simulink model "UAVSlung2"  (R2023a)
settings: Solver=ode45  StartTime=0.0  StopTime=16  RelTol=1e-4
values from neighbouring files (symbols this model uses):
  x0 = [0.1 -0.1 0 0 0 -0.5 2 0 0 0 0 0 0 0 0 0 0 0 0]    [main.m]
settings Model: Creator=KANG  LastModifiedBy=kang
settings DataIOCC: ReturnWorkspaceOutputs=off  TimeSaveName=tout1
settings DebuggingCC: UnconnectedInputMsg=warning  UnconnectedOutputMsg=warning  UnconnectedLineMsg=warning
settings ModelReferenceCC: EnableRefExpFcnMdlSchedulingChecks=on
settings RTWCC: DLArmComputeVersion=19.05

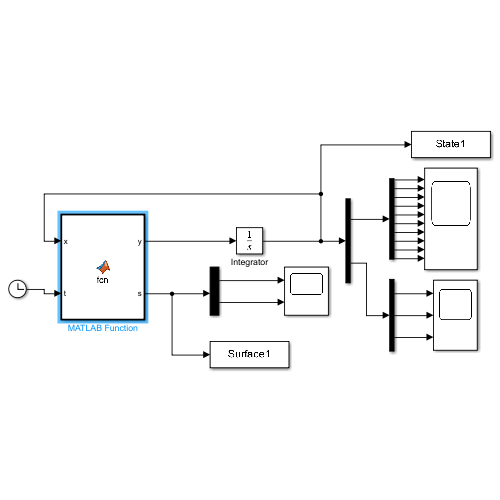
[thumbnail: Simulink's stored preview of the top-level diagram]
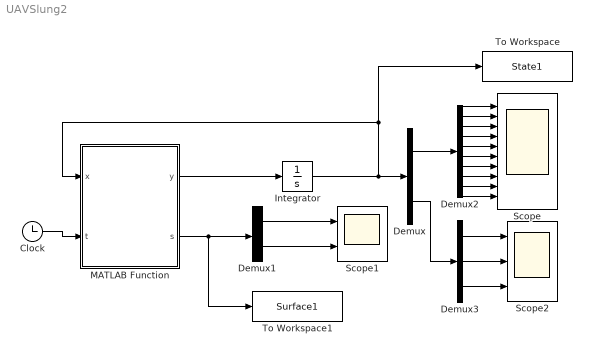
== system UAVSlung2 ==
  Clock : Clock
  Demux : Demux  Outputs=[10,9]
  Demux1 : Demux  Outputs=2
  Demux2 : Demux  Outputs=10
  Demux3 : Demux  Outputs=[-1,-1,-1]
  Integrator : Integrator  InitialCondition=x0
  MATLAB Function : MATLAB Function  TreatAsAtomicUnit=on
  Scope : Scope  NumInputPorts=10
  Scope1 : Scope  NumInputPorts=2
  Scope2 : Scope  NumInputPorts=3
  To Workspace : ToWorkspace  VariableName=State1  SaveFormat=Structure With Time  SampleTime=-1
  To Workspace1 : ToWorkspace  VariableName=Surface1  SaveFormat=Structure With Time  SampleTime=-1
  wires:
  MATLAB Function/1(y) -> Integrator/1
  Clock/1 -> MATLAB Function/2(t)
  MATLAB Function/2(s) -> To Workspace1/1, Demux1/1
  Integrator/1 -> To Workspace/1, MATLAB Function/1(x), Demux/1
  Demux/1 -> Demux2/1
  Demux1/1 -> Scope1/1
  Demux1/2 -> Scope1/2
  Demux2/1 -> Scope/1
  Demux2/2 -> Scope/2
  Demux2/3 -> Scope/3
  Demux2/4 -> Scope/4
  Demux2/5 -> Scope/5
  Demux2/6 -> Scope/6
  Demux2/7 -> Scope/7
  Demux2/8 -> Scope/8
  Demux2/9 -> Scope/9
  Demux2/10 -> Scope/10
  Demux3/1 -> Scope2/1
  Demux3/2 -> Scope2/2
  Demux/2 -> Demux3/1
  Demux3/3 -> Scope2/3

== matlab function UAVSlung2/MATLAB Function ==
  data: x input; y output; t input; s output
function [y, s] = fcn(x, t)
y=zeros(19,1);
s=zeros(9,1);
%% 
%  1-4 theta1 theta2 dtheta1 dtheta2
%  
%  5-10 x y z dx dy dz
%% 
l=0.5; g=9.81; mp=0.5;mq=1.121;
m=mp+mq;


% %% M ,C  G   u 
% M=zeros(5,5);
% M(1,1)=mq+mp;M(2,2)=mq+mp;M(3,3)=mq+mp;M(4,4)=mp*l^2*cos(x(2))^2;M(5,5)=mp*l^2;
% M(1,4)=mp*l*cos(x(1))*cos(x(2));
% M(4,1)=M(1,4);
% M(1,5)=-mp*l*sin(x(1))*sin(x(2));
% M(5,1)=M(1,5);
% M(2,5)=mp*l*cos(x(2));
% M(5,2)=M(2,5);
% M(3,4)=mp*l*sin(x(1))*cos(x(2));
% M(4,3)=M(3,4);
% M(3,5)=mp*l*cos(x(1))*sin(x(2));
% M(5,3)=M(3,5);
% % 
% 
% C=zeros(5,5);
% 
% C(1,4)=-mp*l*x(3)*sin(x(1))*cos(x(2))-mp*l*x(4)*cos(x(1))*sin(x(2));
% C(1,5)=-mp*l*x(3)*cos(x(1))*sin(x(2))-mp*l*x(4)*sin(x(1))*cos(x(2));
% C(2,5)=-mp*l*x(4)*sin(x(2));
% C(3,4)=mp*l*x(3)*cos(x(1))*cos(x(2))-mp*l*x(4)*sin(x(1))*sin(x(2));
% C(3,5)=-mp*l*x(3)*sin(x(1))*sin(x(2))+mp*l*x(4)*cos(x(1))*cos(x(2));
% C(4,4)=-mp*l^2*x(4)*cos(x(2))*sin(x(2));
% C(4,5)=-mp*l^2*x(3)*cos(x(2))*sin(x(2));
% C(5,4)=mp*l^2*x(3)*cos(x(2))*sin(x(2));
% 
% G=[0 0 0 mp*g*l*sin(x(1))*cos(x(2)) mp*g*l*cos(x(1))*sin(x(2))]';




e3=[0 0 1]';


%%

rd=[1,0.5,3];% target point

c11=0.6;c21=0.6;c31=0.6; c12=0;c22=0;c32=0; % gains for sliding mode manifold 

Sx=c11*(x(5)-rd(1))+x(8)-c12*sin(x(1))*cos(x(2));
Sy=c21*(x(6)-rd(2))+x(9)-c22*sin(x(2));
Sz=c31*(x(7)-rd(3))+x(10)+c32-c32*cos(x(1))*cos(x(2));

d=0.1*[1*sin(t),2*sin(t),1*sin(t)]';  % disturbances



k11=0;k21=0;k31=0; k12=2;k22=2;k32=2;% control gains
%% controller
vx1=-k11*(Sx)-k12*sig(Sx,0.5)+1*x(11)-x(17);
vy1=-k21*(Sy)-k22*sig(Sy,0.5)+1*x(12)-x(18);
vz1=-k31*(Sz)-k32*sig(Sz,0.5)+1*x(13)-x(19);

vx=-c11*x(8)+c12*(cos(x(1))*cos(x(2))*x(3)-sin(x(1))*sin(x(2))*x(4))+vx1;
vy=-c21*x(9)+c22*cos(x(2))*x(4)+vy1;
vz=-c31*x(10)-c32*(sin(x(1))*cos(x(2))*x(3)+cos(x(1))*sin(x(2))*x(4))+vz1;


%*******
%  11-13 super twisting controller
y(11)=-1*sign(Sx);
y(12)=-1*sign(Sy);
y(13)=-1*sign(Sz);

%% super twisting observer 
%14-16 estimation of sliding manifold
%17-19 estimation of disturbance

lam1=-1.5*5^0.5*sig(x(14)-Sx,0.5)+x(17);
lam2=-1.5*5^0.5*sig(x(15)-Sy,0.5)+x(18);
lam3=-1.5*5^0.5*sig(x(16)-Sz,0.5)+x(19);

y(14)=vx+lam1;
y(15)=vy+lam2;
y(16)=vz+lam3;



y(17)=-1.1*5*sign(x(17)-lam1);
y(18)=-1.1*5*sign(x(18)-lam2);
y(19)=-1.1*5*sign(x(19)-lam3);


M1=[m-mp+mp*sin(x(1))^2*cos(x(2))^2,mp*sin(x(1))*sin(x(2))*cos(x(2)),-mp*sin(x(1))*cos(x(1))*cos(x(2))^2;...
    mp*sin(x(1))*sin(x(2))*cos(x(2)),m-mp*cos(x(2))^2,-mp*sin(x(2))*cos(x(1))*cos(x(2));...
    -mp*sin(x(1))*cos(x(1))*cos(x(2))^2,-mp*sin(x(2))*cos(x(1))*cos(x(2)),m-mp+mp*cos(x(1))^2*cos(x(2))^2];

y(5:7)=x(8:10); 

y(8:10)=[vx;vy;vz]+M1\d;


% f=[-mp*l*(sin(u(1))*cos(u(2))*u(3)^2+2*sin(u(2))*cos(u(1))*u(3)*u(4)+sin(u(1))*sin(u(2))*u(4)^2);...
%    -mp*l*(sin(u(2))*u(4)^2;...
%     mp*l*(cos(u(1))*cos(u(2))*u(3)^2-2*sin(u(2))*sin(u(1))*u(3)*u(4)+cos(u(1))*cos(u(2))*u(4)^2)];

f=[mp*(-g*sin(x(1))*cos(x(1))*cos(x(2))^3-sin(x(1))*cos(x(2))*l*x(3)^2-sin(x(1))*sin(x(2))*l*x(4)^2);...
   mp*(-l*cos(x(2))^2*x(3)^2-g*cos(x(1))*cos(x(2))-l*x(4)^2)*sin(x(2));...
   mp*(-g+g*cos(x(1))^2*cos(x(2))^2+l*cos(x(1))*cos(x(2))^3*x(3)^2+l*cos(x(1))*cos(x(2))*x(4)^2)];
%%
U=M1*[vx;vy;vz]+f+m*g*e3;

% dy=M\(-C*[x(8:10);x(3:4)]-G+[U-m*g*e3+d;0;0]); 
% y(3:4)=dy(4:5);
% y(8:10)=dy(1:3);

F1=y(8);
F2=y(9);
F3=y(10);

y(1)=x(3);
y(2)=x(4);
y(3)=(2*l*sin(x(2))*x(3)*x(4)-g*sin(x(1))-F1*cos(x(1))-F3*sin(x(1)))/(l*cos(x(2)));
y(4)=(F1*sin(x(1))*sin(x(2))-F2*cos(x(2))-F3*cos(x(1))*sin(x(2))-l*sin(x(2))*cos(x(2))*x(3)^2-g*cos(x(1))*sin(x(2)))/l;

s(1)=Sx;
s(2)=Sy;
s(3)=Sz;



psaid=0;
phid=asin((U(1)*sin(psaid)-U(2)*cos(psaid))/norm(U));
thetad=atan((U(1)*cos(psaid)+U(2)*sin(psaid))/U(3));
s(4)=phid;
s(5)=thetad;
% s(5)=norm(y(8:10));
s(6)=norm(U);
s(7:9)=U;

end
